simulink model "Engine_Model"  (R2016b)
settings: Solver=VariableStepAuto  StartTime=0.0  StopTime=10.0  RelTol=1e-3
undefined symbols (not defined in the file or in its folder): EngMdl
libraries: gtlink2017rt x1
settings Model: Creator=r03schne  LastModifiedBy=r03schne

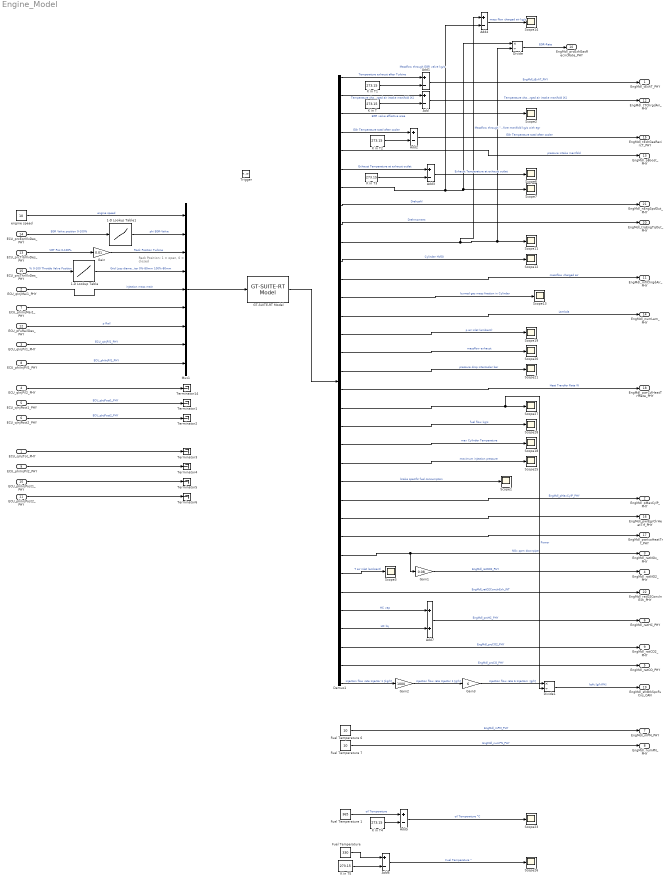
== system Engine_Model ==
  note: Rack Position: 1 = open,
      | 			  0 = closed
  ECU_qInjTot_PHY : Inport
  ECU_qInjMai1_PHY : Inport  Port=2
  ECU_qInjPil1_PHY : Inport  Port=3
  ECU_qInjPil2_PHY : Inport  Port=4
  ECU_qInjPost1_PHY : Inport  Port=5
  ECU_qInjPost2_PHY : Inport  Port=6
  ECU_phiInjMai1_PHY : Inport  Port=7
  ECU_phiInjPil1_PHY : Inport  Port=8
  ECU_phiInjPil2_PHY : Inport  Port=9
  ECU_phiInjPost1_PHY : Inport  Port=10
  ECU_phiInjPost2_PHY : Inport  Port=11
  ECU_pFuRailDes_PHY : Inport  Port=12
  ECU_prcTrbVlvDes_PHY : Inport  Port=13
  ECU_prcEgrVlvDes_PHY : Inport  Port=14
  ECU_prcThrVlvDes_PHY : Inport  Port=15
  Trigger : TriggerPort  TriggerType=function-call  VariantControl=Variant  SampleTimeType=periodic  SampleTime=EngMdl.tiSimnTiStep_C.Value  PortDimensions=1
  1-D Lookup Table : Lookup_n-D  NumberOfTableDimensions=1  BreakpointsForDimension1=[0 100]  Table=[80 0]  InternalRulePriority=Speed  RndMeth=Simplest  InputSameDT=on
  1-D Lookup Table1 : Lookup_n-D  NumberOfTableDimensions=1  BreakpointsForDimension1=[0 100]  Table=[0 90]  InternalRulePriority=Speed  RndMeth=Simplest  InputSameDT=on
  Add{,1..6} (7 alike) : Sum  Inputs=+-
  Add7 : Sum
  Demux1 : Demux  Outputs=34
  Divide : Product  Inputs=*/
  Divide1 : Product  Inputs=*/
  "Fuel Temperature " : Constant  Value=330
  Fuel Temperature 1 : Constant  Value=365
  Fuel Temperature 6 : Constant  Value=10
  Fuel Temperature 7 : Constant  Value=10
  GT-SUITE-RT Model : gtlink2017rt/GT-SUITE-RT Model  gti_fname=OptiTruck_RT_enginemodel_v0  gti_dur=SIMULINK  gti_msg=No runtime messages  gti_dt=EngMdl.tiSimnTiStep_C.Value  gti_ni=9  gti_no=34  gti_parnam='ign'  gti_parval='ign'  gti_cylnam='ign'  gti_nrtpr=-1
      settings: AttributesFormatString=(%<gti_fname>.dat)
  Gain : Gain  Gain=0.01
  Gain1 : Gain  Gain=0.08
  Gain2 : Gain  Gain=1000
  Gain3 : Gain  Gain=6
  K in T{,1..5} (6 alike) : Constant  Value=273.15
  Mux1 : Mux  Inputs=9
  Scope{1..3,6..7,11..14,18..21,23,25..28} (18 alike) : Scope
  Terminator{1..6,14} (7 alike) : Terminator
  engine speed : Constant  Value=10
  EngMdl_tExhT_PHY : Outport
  EngMdl_pMaxCylP_PHY : Outport  Port=2
  EngMdl_ratNOx_PHY : Outport  Port=3
  EngMdl_ratNO2_PHY : Outport  Port=4
  EngMdl_ratCO_PHY : Outport  Port=5
  EngMdl_ratHC_PHY : Outport  Port=6
  EngMdl_mPM_PHY : Outport  Port=7
  EngMdl_numPN_PHY : Outport  Port=8
  EngMdl_ratCO2_PHY : Outport  Port=9
  EngMdl_prcExhGasRecircRate_PHY : Outport  Port=10
  EngMdl_mflChrgdAir_PHY : Outport  Port=11
  EngMdl_tTChrgdAir_PHY : Outport  Port=12
  EngMdl_pBoost_PHY : Outport  Port=13
  EngMdl_numLam_PHY : Outport  Port=14
  EngMdl_tExhGasRecircT_PHY : Outport  Port=15
  EngMdl_pwrEgrClrHeatTrf_PHY : Outport  Port=16
  EngMdl_pwrIcoHeatTrf_PHY : Outport  Port=17
  EngMdl_pwrCylHeatTrfRate_PHY : Outport  Port=18
  EngMdl_sfcBrkSpcFuCns_CAN : Outport  Port=19
  EngMdl_trqEngTqOut_PHY : Outport  Port=20
  EngMdl_nEngSpdOut_PHY : Outport  Port=21
  EngMdl_ratO2ConcInExh_PHY : Outport  Port=22
  wires:
  GT-SUITE-RT Model/1 -> Demux1/1
  Mux1/1 -> GT-SUITE-RT Model/1
  Demux1/1 -> Add1/1  "Temperature exhaust after Turbine"
  engine speed/1 -> Mux1/1  "engine speed"
  ECU_prcEgrVlvDes_PHY/1 -> 1-D Lookup Table1/1  "EGR Valve position 0-100%"
  Demux1/2 -> Add/1  "Temperature charged air intake manifold [K]"
  Demux1/3 -> Scope2/1  "EGR valve effective area"
  Demux1/4 -> Add2/1  "EGr Temperature total after cooler"
  Demux1/5 -> EngMdl_pBoost_PHY/1  "pressure intake manifold"
  Demux1/7 -> Add4/2, Divide/1, Scope7/1  "Massflow through EGR valve kg/s"
  Add/1 -> EngMdl_tTChrgdAir_PHY/1  "Temperature charged air intake manifold [K]"
  K in T/1 -> Add/2
  K in T1/1 -> Add1/2
  Demux1/9 -> EngMdl_trqEngTqOut_PHY/1  "Drehmoment"
  Demux1/8 -> EngMdl_nEngSpdOut_PHY/1  "Drehzahl"
  Add2/1 -> EngMdl_tExhGasRecircT_PHY/1  "EGr Temperature total after cooler"
  K in T2/1 -> Add2/2
  Add3/1 -> Scope6/1  "Exhaust Temperature at exhaust outlet"
  K in T3/1 -> Add3/2
  Demux1/6 -> Add3/1  "Exhaust Temperature at exhaust outlet"
  Demux1/10 -> Add4/1, Divide/2, Scope11/1  "Massflow through \"grid loss\" before manifold kg/s with egr"
  Gain/1 -> Mux1/3  "Rack Position Turbine"
  ECU_qInjMai1_PHY/1 -> Mux1/5  "injection mass main"
  Demux1/11 -> Scope12/1  "Cylinder HV50"
  ECU_pFuRailDes_PHY/1 -> Mux1/7  "p Rail"
  1-D Lookup Table/1 -> Mux1/4  "Grid Loss diameter 0%-80mm 100%-80mm"
  Divide/1 -> EngMdl_prcExhGasRecircRate_PHY/1  "EGR-Rate"
  Add4/1 -> Scope14/1  "mass flow charged air kg/s"
  Demux1/12 -> EngMdl_mflChrgdAir_PHY/1  "massflow charged air"
  Demux1/13 -> Scope13/1  "burned gas mass fraction in Cylinder"
  Demux1/14 -> EngMdl_numLam_PHY/1  "Lambda"
  Demux1/21 -> Scope18/1  "max Cylinder Temperature"
  Demux1/15 -> Scope19/1  "p air inlet (ambient)"
  Demux1/16 -> Scope20/1  "massflow exhaust"
  Demux1/17 -> Scope21/1  "pressure drop intercooler bar"
  Demux1/18 -> EngMdl_pwrCylHeatTrfRate_PHY/1  "Heat Transfer Rate W"
  Demux1/23 -> Scope1/1  "brake specific fuel consumption"
  Fuel Temperature 1/1 -> Add5/1  "oil Temperature"
  Demux1/22 -> Scope25/1  "maximum injection pressure"
  K in T4/1 -> Add5/2
  Add5/1 -> Scope23/1  "oil Temperature °C"
  "Fuel Temperature "/1 -> Add6/1
  K in T5/1 -> Add6/2
  Add6/1 -> Scope26/1  "Fuel Temperature °"
  Demux1/19 -> Divide1/2, Scope27/1  "Power"
  Demux1/20 -> Scope28/1  "fuel flow kg/s"
  ECU_qInjPil1_PHY/1 -> Mux1/8  "ECU_qInjPil1_PHY"
  ECU_qInjPil2_PHY/1 -> Terminator14/1
  ECU_qInjPost1_PHY/1 -> Terminator1/1  "ECU_qInjPost1_PHY"
  ECU_qInjPost2_PHY/1 -> Terminator2/1  "ECU_qInjPost2_PHY"
  ECU_phiInjMai1_PHY/1 -> Mux1/6
  ECU_phiInjPil1_PHY/1 -> Mux1/9  "ECU_phiInjPil1_PHY"
  ECU_phiInjPil2_PHY/1 -> Terminator4/1
  ECU_phiInjPost1_PHY/1 -> Terminator5/1
  ECU_prcTrbVlvDes_PHY/1 -> Gain/1  "VGT Pos 0-100%"
  ECU_prcThrVlvDes_PHY/1 -> 1-D Lookup Table/1  "% 0-100 Throttle Valve Position"
  1-D Lookup Table1/1 -> Mux1/2  "phi EGR-Valve"
  Add1/1 -> EngMdl_tExhT_PHY/1  "EngMdl_tExhT_PHY"
  Demux1/24 -> EngMdl_pMaxCylP_PHY/1  "EngMdl_pMaxCylP_PHY"
  Gain1/1 -> EngMdl_ratNO2_PHY/1  "EngMdl_ratNO2_PHY"
  Demux1/33 -> EngMdl_ratCO_PHY/1  "EngMdl_prcCO_PHY"
  Add7/1 -> EngMdl_ratHC_PHY/1  "EngMdl_prcHC_PHY"
  Fuel Temperature 6/1 -> EngMdl_mPM_PHY/1  "EngMdl_mPM_PHY"
  Demux1/32 -> EngMdl_ratCO2_PHY/1  "EngMdl_prcCO2_PHY"
  Fuel Temperature 7/1 -> EngMdl_numPN_PHY/1  "EngMdl_numPN_PHY"
  ECU_phiInjPost2_PHY/1 -> Terminator6/1
  Demux1/25 -> EngMdl_pwrEgrClrHeatTrf_PHY/1
  Demux1/26 -> EngMdl_pwrIcoHeatTrf_PHY/1
  ECU_qInjTot_PHY/1 -> Terminator3/1
  Demux1/29 -> EngMdl_ratO2ConcInExh_PHY/1  "EngMdl_ratO2ConcInExh_INT"
  Demux1/27 -> Gain1/1, EngMdl_ratNOx_PHY/1  "NOx ppm downpipe"
  Demux1/28 -> Scope3/1  "T air inlet (ambient)"
  Demux1/30 -> Add7/1  "HC vap"
  Demux1/31 -> Add7/2  "HC liq"
  Demux1/34 -> Gain2/1  "injection flow rate Injector 1 [kg/h]"
  Gain2/1 -> Gain3/1  "injection flow rate Injector 1 [g/h]"
  Gain3/1 -> Divide1/1  "injection flow rate 6 Injectors  [g/h]"
  Divide1/1 -> EngMdl_sfcBrkSpcFuCns_CAN/1  "bsfc [g/kWh]"
